simulink model "TrafficLight_SF_Topic3_Task3"  (R2019a)
settings: Solver=FixedStepDiscrete  StartTime=0.0  StopTime=Inf  RelTol=1e-3
settings Model: EnablePacing=on  Creator=Raouf  LastModifiedBy=Raouf
settings OptimizationCC: DefaultParameterBehavior=Inlined  EnhancedBackFolding=on  PassReuseOutputArgsAs=Individual arguments  OptimizeBlockOrder=speed  DifferentSizesBufferReuse=on  OptimizationCustomize=off
settings DebuggingCC: ParameterTunabilityLossMsg=error
settings SFSimCC: MATLABDynamicMemAlloc=off
settings RTWCC: SystemTargetFile=ert.tlc  GenCodeOnly=on  TemplateMakefile=ert_default_tmf  GenerateReport=on  IncludeHyperlinkInReport=on  LaunchReport=on  GenerateTraceInfo=on  GenerateTraceReport=on  GenerateTraceReportSl=on  GenerateTraceReportSf=on  GenerateTraceReportEml=on
settings CodeAppCC: ForceParamTrailComments=on  IgnoreCustomStorageClasses=off  OperatorAnnotations=on  SimulinkDataObjDesc=on  SFDataObjDesc=on  InsertBlockDesc=on
settings ERTTargetCC: TargetLangStandard=C99 (ISO)  GenerateSampleERTMain=on  InlinedParameterPlacement=NonHierarchical  ERTCustomFileTemplate=example_file_process.tlc

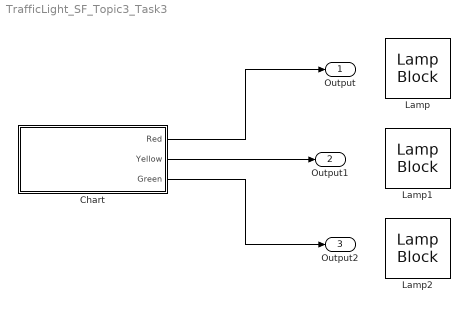
== system TrafficLight_SF_Topic3_Task3 ==
  Chart : Stateflow chart  BlockKeywords=__PRM__SERIALIZED__DATA__:Stateflow Chart,Stateflow Diagram  TreatAsAtomicUnit=on
  Lamp : LampBlock
  Lamp1 : LampBlock
  Lamp2 : LampBlock
  Output : Outport
  Output1 : Outport  Port=2
  Output2 : Outport  Port=3
  wires:
  Chart/1(Red) -> Output/1
  Chart/2(Yellow) -> Output1/1
  Chart/3(Green) -> Output2/1

== stateflow chart TrafficLight_SF_Topic3_Task3/Chart ==
  state Stop
    en:
    Red = 0;
    Yellow = 0;
    Green = 0;
    du:
    Red = 1;
    Yellow = 0;
    Green = 0;
    exit:
    Red = 0;
    Yellow = 0;
    Green = 0;
  state Ready
    en:
    du:
    Red = 0;
    Yellow = 1;
    Green = 0;
    exit:
    Red = 0;
    Yellow = 0;
    Green = 0;
  state Go
    en:
    du:
    Red = 0;
    Yellow = 0;
    Green = 1;
    exit:
    Red = 0;
    Yellow = 0;
    Green = 1;
  (default) -> Stop
  Stop -> Ready : after(5,sec)
  Ready -> Go : after(2,sec)
  Go -> Stop : after(10,sec)
  data: Red output boolean; Yellow output boolean; Green output boolean
